simulink model "innerflow"  (R2023a)
settings: Solver=ode45  StartTime=0.0  StopTime=inf  RelTol=1e-3  EnableMultiTasking=on
settings Model: Creator=wkmiao  LastModifiedBy=wkmiao
settings SolverCC: AlgebraicLoopSolver=TrustRegion
settings DataIOCC: LimitDataPoints=on  SaveFormat=Array  SignalLoggingSaveFormat=ModelDataLogs  ReturnWorkspaceOutputs=off
settings OptimizationCC: InitFltsAndDblsToZero=on  LifeSpan=inf
settings DebuggingCC: SaveWithParameterizedLinksMsg=none  UnderspecifiedInitializationDetection=Classic  MergeDetectMultiDrivingBlocksExec=none  SignalResolutionControl=TryResolveAllWithWarning  SolverPrmCheckMsg=warning  MultiTaskDSMMsg=warning  MultiTaskCondExecSysMsg=none  FcnCallInpInsideContextMsg=warning  UnconnectedInputMsg=warning  UnconnectedOutputMsg=warning  UnconnectedLineMsg=warning  SFUnexpectedBacktrackingDiag=warning  SFNoUnconditionalDefaultTransitionDiag=warning  SFExecutionAtInitializationDiag=none  ArithmeticOperatorsInVariantConditions=warning
settings HardwareCC: ProdBitPerPointer=32  ProdBitPerSizeT=32  ProdBitPerPtrDiffT=32  ProdLargestAtomicFloat=None  ProdIntDivRoundTo=Undefined  ProdEndianess=Unspecified  ProdWordSize=32  ProdHWDeviceType=32-bit Generic
settings ModelReferenceCC: PropagateSignalLabelsOutOfModel=off
settings SFSimCC: SimParseCustomCode=off
settings CodeAppCC: StateflowObjectComments=on
settings GRTTargetCC: TargetFcnLib=ansi_tfl_tmw.mat  TargetLangStandard=C89/C90 (ANSI)  CombineOutputUpdateFcns=off  GRTInterface=on
settings ConfigComp: CovMetricSettings=dw  CovSaveCumulativeToWorkspaceVar=on  CovSaveSingleToWorkspaceVar=on

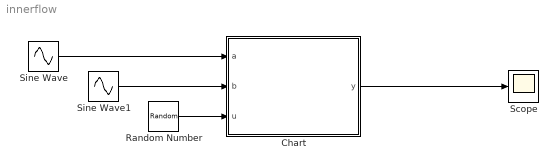
== system innerflow ==
  Chart : Stateflow chart  TreatAsAtomicUnit=on
  Random Number : RandomNumber  SampleTime=0
  Scope : Scope
  Sine Wave : Sin  SampleTime=0
  Sine Wave1 : Sin  Frequency=1.5  Phase=-1  SampleTime=0
  wires:
  Chart/1(y) -> Scope/1
  Sine Wave/1 -> Chart/1(a)
  Sine Wave1/1 -> Chart/2(b)
  Random Number/1 -> Chart/3(u)

== stateflow chart innerflow/Chart ==
  state B
    entry:printf("act1 \n\n");
    du:printf("\n\n act2 \n\n");
    (default) -> (junction 21) : {printf("\n\n act3 \n\n");}
    B -> (junction 21) [order 1] : {printf("\n\n act4 \n\n");}
    (junction 21) -> (junction 22) [order 1] : [a > 0]
    (junction 21) -> (junction 23) [order 2] : {
        | y = 0;
        | }
    (junction 22) -> (junction 24) : {
        | y = u;
        | }
    (junction 24) -> (junction 23)
  state A
    (default) -> (junction 17)
    (junction 17) -> (junction 19) [order 1] : [a > 0]
    (junction 17) -> (junction 18) [order 2] : {
        | y = -1;
        | }
    (junction 19) -> (junction 20) : {
        | y = 1;
        | }
    (junction 20) -> (junction 18)
  (default) -> A
  A -> B : [b > 0]
  B -> A [order 1] : [b < 0]
  data: a input; b input; u input; y output double =0
